simulink model "Motor_Dynamics"  (R2021a)
settings: Solver=VariableStepAuto  StartTime=0.0  StopTime=10  FixedStep=.001  MaxStep=0.001  RelTol=1e-4
values from neighbouring files (symbols this model uses):
  b_m = 2.415e-6    (= 2.415e-06)    [MotorDynamics.m]
  Jr = 6.5*10^(-7)    (= 6.5e-07)    [MotorDynamics.m]
  Kemf = 0.00255    [MotorDynamics.m]
  Kt = median((-Data(:,9)./(Data(:,12))))    [MotorDynamics.m]
  L = 0.001*R    (= 0.000117)    [MotorDynamics.m]
  R = 0.117    [MotorDynamics.m]
settings Model: Creator=Nicky  LastModifiedBy=YeBobo
settings SolverCC: ZeroCrossAlgorithm=Adaptive  AlgebraicLoopSolver=LineSearch
settings DataIOCC: ReturnWorkspaceOutputs=off
settings DebuggingCC: SFMachineParentedDataDiag=warning  ArithmeticOperatorsInVariantConditions=warning
settings SFSimCC: SimUseLocalCustomCode=off  CustomCodeUndefinedFunction=UseInterfaceOnly
settings RTWCC: RTWUseLocalCustomCode=off

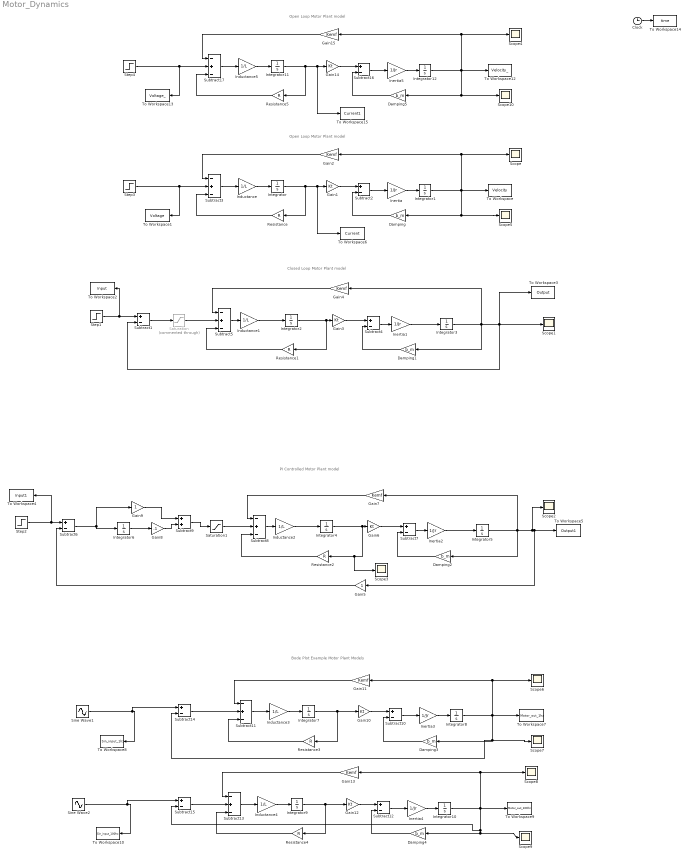
== system Motor_Dynamics ==
  note: Open Loop Motor Plant model
  note: Closed Loop Motor Plant model
  note: PI Controlled Motor Plant model
  note: Bode Plot Example Motor Plant Models
  note: Open Loop Motor Plant model
  Clock : Clock
  Damping{,1..5} (6 alike) : Gain  Gain=b_m
  Gain{1,3,6,10,12,14} (6 alike) : Gain  Gain=Kt
  Gain{2,4,7,11,13,15} (6 alike) : Gain  Gain=Kemf
  Gain5 : Gain
  Gain8 : Gain  Gain=.1
  Gain9 : Gain
  Inductance{,1..5} (6 alike) : Gain  Gain=1/L
  Inertia{,1..5} (6 alike) : Gain  Gain=1/Jr
  Integrator{,1..5,7..12} (12 alike) : Integrator  LimitOutput=on  LowerSaturationLimit=0
  Integrator6 : Integrator
  Resistance{,1..5} (6 alike) : Gain  Gain=R
  Saturation : Saturate  Commented=through  UpperLimit=12  LowerLimit=0  LinearizeAsGain=off
  Saturation1 : Saturate  UpperLimit=12  LowerLimit=0  LinearizeAsGain=off
  Scope{,1..10} (11 alike) : Scope
  Sine Wave1 : Sin  Amplitude=100  Bias=2000  SampleTime=0
  Sine Wave2 : Sin  Amplitude=100  Bias=2000  Frequency=1000  SampleTime=0
  Step1 : Step  Time=0  After=1000
  Step2 : Step  Time=2  Before=1000  After=500  SampleTime=0
  Step3 : Step  Time=0  SampleTime=0
  Step4 : Step  Time=0  SampleTime=0
  Subtract{1..2,4,6..7,10,12,14..16} (10 alike) : Sum  Inputs=+-
  Subtract{3,5,8,11,13,17} (6 alike) : Sum  Inputs=-+-
  Subtract9 : Sum
  To Workspace : ToWorkspace  VariableName=Velocity  SampleTime=-1
      settings: Save2DSignal=2-D array (concatenate along first dimension)
  To Workspace1 : ToWorkspace  VariableName=Voltage  SampleTime=-1
      settings: Save2DSignal=2-D array (concatenate along first dimension)
  To Workspace10 : ToWorkspace  VariableName=Sin_input_100hz  SampleTime=-1
      settings: Save2DSignal=2-D array (concatenate along first dimension)
  To Workspace12 : ToWorkspace  VariableName=Velocity_  SampleTime=0.0001
      settings: Save2DSignal=2-D array (concatenate along first dimension)
  To Workspace13 : ToWorkspace  VariableName=Voltage_  SampleTime=0.0001
      settings: Save2DSignal=2-D array (concatenate along first dimension)
  To Workspace14 : ToWorkspace  VariableName=time  SampleTime=-1
      settings: Save2DSignal=2-D array (concatenate along first dimension)
  To Workspace15 : ToWorkspace  VariableName=Current1  SampleTime=-1
      settings: Save2DSignal=2-D array (concatenate along first dimension)
  To Workspace2 : ToWorkspace  VariableName=Input  SampleTime=0.0001
      settings: Save2DSignal=2-D array (concatenate along first dimension)
  To Workspace3 : ToWorkspace  VariableName=Output  SampleTime=0.0001
      settings: Save2DSignal=2-D array (concatenate along first dimension)
  To Workspace4 : ToWorkspace  VariableName=Input1  SampleTime=-1
      settings: Save2DSignal=2-D array (concatenate along first dimension)
  To Workspace5 : ToWorkspace  VariableName=Output1  SampleTime=-1
      settings: Save2DSignal=2-D array (concatenate along first dimension)
  To Workspace6 : ToWorkspace  VariableName=Current  SampleTime=-1
      settings: Save2DSignal=2-D array (concatenate along first dimension)
  To Workspace7 : ToWorkspace  VariableName=Motor_out_1hz  SampleTime=-1
      settings: Save2DSignal=2-D array (concatenate along first dimension)
  To Workspace8 : ToWorkspace  VariableName=Sin_input_1hz  SampleTime=-1
      settings: Save2DSignal=2-D array (concatenate along first dimension)
  To Workspace9 : ToWorkspace  VariableName=Motor_out_100hz  SampleTime=-1
      settings: Save2DSignal=2-D array (concatenate along first dimension)
  wires:
  Clock/1 -> To Workspace14/1
  Subtract3/1 -> Inductance/1
  Inductance/1 -> Integrator/1
  Gain1/1 -> Subtract2/1
  Subtract2/1 -> Inertia/1
  Damping/1 -> Subtract2/2
  Resistance/1 -> Subtract3/3
  Gain2/1 -> Subtract3/1
  Inductance1/1 -> Integrator2/1
  Subtract5/1 -> Inductance1/1
  Gain4/1 -> Subtract5/1
  Damping1/1 -> Subtract4/2
  Resistance1/1 -> Subtract5/3
  Subtract4/1 -> Inertia1/1
  Inertia1/1 -> Integrator3/1
  Gain3/1 -> Subtract4/1
  Saturation/1 -> Subtract5/2
  Inertia/1 -> Integrator1/1
  Integrator2/1 -> Gain3/1, Resistance1/1
  Integrator/1 -> To Workspace6/1, Gain1/1, Resistance/1
  Step3/1 -> To Workspace1/1, Subtract3/2
  Step1/1 -> To Workspace2/1, Subtract1/1
  Integrator3/1 -> Subtract1/2, To Workspace3/1, Scope1/1, Damping1/1, Gain4/1
  Damping2/1 -> Subtract7/2
  Subtract8/1 -> Inductance2/1
  Resistance2/1 -> Subtract8/3
  Subtract7/1 -> Inertia2/1
  Gain7/1 -> Subtract8/1
  Inductance2/1 -> Integrator4/1
  Gain6/1 -> Subtract7/1
  Integrator4/1 -> Gain6/1, Scope3/1, Resistance2/1
  Saturation1/1 -> Subtract8/2
  Inertia2/1 -> Integrator5/1
  Integrator5/1 -> Scope2/1, Gain5/1, To Workspace5/1, Damping2/1, Gain7/1
  Integrator1/1 -> Gain2/1, Scope/1, Scope5/1, Damping/1, To Workspace/1
  Gain5/1 -> Subtract6/2
  Subtract1/1 -> Saturation/1
  Integrator6/1 -> Gain8/1
  Subtract6/1 -> Gain9/1, Integrator6/1
  Subtract9/1 -> Saturation1/1
  Gain9/1 -> Subtract9/1
  Gain8/1 -> Subtract9/2
  Step2/1 -> To Workspace4/1, Subtract6/1
  Inertia3/1 -> Integrator8/1
  Subtract10/1 -> Inertia3/1
  Gain11/1 -> Subtract11/1
  Resistance3/1 -> Subtract11/3
  Integrator8/1 -> Gain11/1, Scope6/1, Subtract14/2, Scope7/1, Damping3/1, To Workspace7/1
  Damping3/1 -> Subtract10/2
  Gain10/1 -> Subtract10/1
  Subtract11/1 -> Inductance3/1
  Inductance3/1 -> Integrator7/1
  Sine Wave1/1 -> Subtract14/1, To Workspace8/1
  Integrator7/1 -> Gain10/1, Resistance3/1
  Integrator10/1 -> Gain13/1, Scope8/1, Subtract15/2, Scope9/1, Damping4/1, To Workspace9/1
  Damping4/1 -> Subtract12/2
  Gain12/1 -> Subtract12/1
  Resistance4/1 -> Subtract13/3
  Integrator9/1 -> Gain12/1, Resistance4/1
  Subtract13/1 -> Inductance4/1
  Inductance4/1 -> Integrator9/1
  Sine Wave2/1 -> Subtract15/1, To Workspace10/1
  Gain13/1 -> Subtract13/1
  Inertia4/1 -> Integrator10/1
  Subtract12/1 -> Inertia4/1
  Subtract14/1 -> Subtract11/2
  Subtract15/1 -> Subtract13/2
  Inductance5/1 -> Integrator11/1
  Step4/1 -> To Workspace13/1, Subtract17/2
  Integrator12/1 -> Gain15/1, Scope4/1, Scope10/1, Damping5/1, To Workspace12/1
  Damping5/1 -> Subtract16/2
  Resistance5/1 -> Subtract17/3
  Integrator11/1 -> To Workspace15/1, Gain14/1, Resistance5/1
  Gain15/1 -> Subtract17/1
  Inertia5/1 -> Integrator12/1
  Subtract16/1 -> Inertia5/1
  Gain14/1 -> Subtract16/1
  Subtract17/1 -> Inductance5/1
